simulink model "problem5"  (R2020a)
settings: Solver=VariableStepAuto  StartTime=0.0  StopTime=10.0  RelTol=1e-3
undefined symbols (not defined in the file): c, R
settings Model: Creator=Riyansh  LastModifiedBy=Riyansh

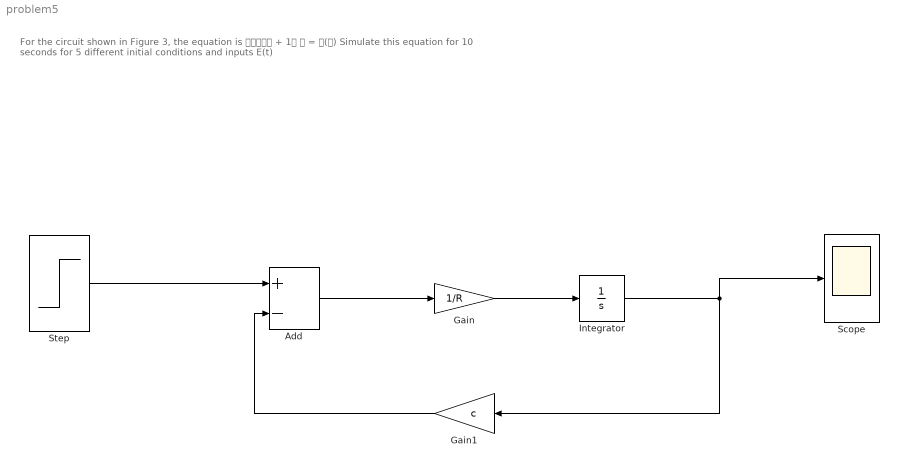
== system problem5 ==
  note: For the circuit shown in Figure 3, the equation is 𝑅𝑑𝑄𝑑𝑡 + 1𝐶 𝑄 = 𝐸(𝑡)
      | Simulate this equation for 10 seconds for 5 different initial conditions and inputs E(t)
  Add : Sum  Inputs=+-
  Gain : Gain  Gain=1/R
  Gain1 : Gain  Gain=c
  Integrator : Integrator  InitialCondition=5
  Scope : Scope
  Step : Step  SampleTime=0
  wires:
  Gain1/1 -> Add/2
  Add/1 -> Gain/1
  Integrator/1 -> Scope/1, Gain1/1
  Gain/1 -> Integrator/1
  Step/1 -> Add/1
